simulink model "short_transmission_line_design"  (R2014b)
settings: Solver=ode23tb  StartTime=0.0  StopTime=1  RelTol=1e-3
libraries: powerlib x6, powerlib_meascontrol x6
settings Model: Creator=Amr Saleh  LastModifiedBy=Amr Saleh

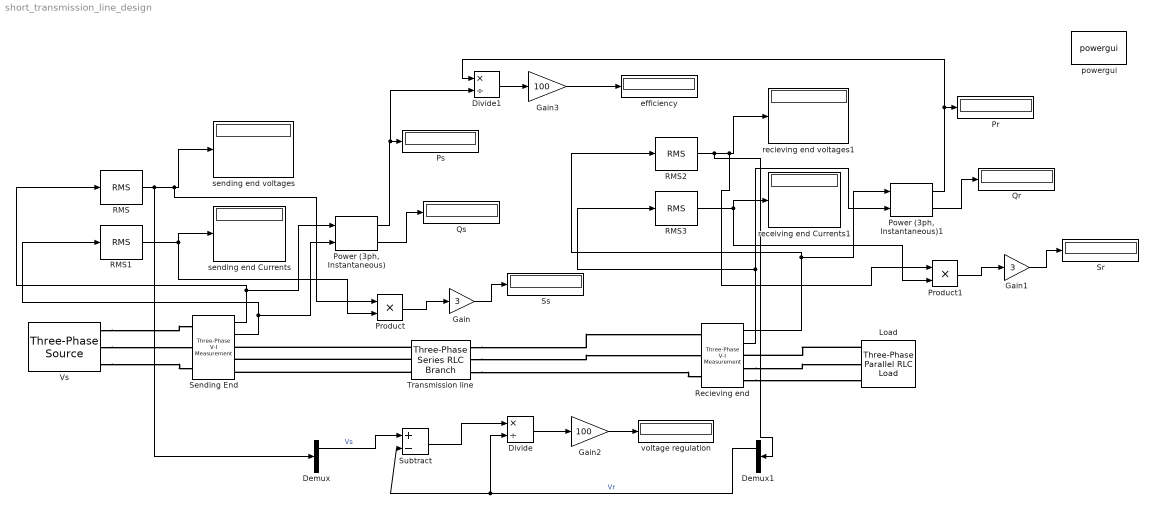
== system short_transmission_line_design ==
  Demux : Demux  Outputs=3
  Demux1 : Demux  Outputs=3
  Divide : Product  Inputs=*/
  Divide1 : Product  Inputs=*/
  Gain : Gain  Gain=3
  Gain1 : Gain  Gain=3
  Gain2 : Gain  Gain=100
  Gain3 : Gain  Gain=100
  Load : powerlib/Elements/Three-Phase Parallel RLC Load  LConnTagsString=A|B|C  Configuration=Y (grounded)  NominalVoltage=220e3  NominalFrequency=60  ActivePower=304.8e6  InductivePower=228.6e6  CapacitivePower=0  Measurements=None  LoadType=constant Z
  "Power (3ph, Instantaneous)" : powerlib_meascontrol/Measurements/Power (3ph, Instantaneous)
  "Power (3ph, Instantaneous)1" : powerlib_meascontrol/Measurements/Power (3ph, Instantaneous)
  Pr : Display
  Product : Product
  Product1 : Product
  Ps : Display
  Qr : Display
  Qs : Display
  RMS{,1..3} (4 alike) : powerlib_meascontrol/Measurements/RMS  TrueRMS=on  Freq=60  RMSInit=0  Ts=0
  Recieving end : powerlib/Measurements/Three-Phase V-I Measurement  VoltageMeasurement=phase-to-ground  SetLabelV=off  LabelV=Vabc  Vpu=off  VpuLL=off  CurrentMeasurement=yes  SetLabelI=off  LabelI=Iabc  Ipu=off  Pbase=100e6  Vbase=500e3  OutputType=Complex  PhasorSimulation=off  PSBequivalent=0
  Sending End : powerlib/Measurements/Three-Phase V-I Measurement  VoltageMeasurement=phase-to-ground  SetLabelV=off  LabelV=Vabc  Vpu=off  VpuLL=off  CurrentMeasurement=yes  SetLabelI=off  LabelI=Iabc  Ipu=off  Pbase=100e6  Vbase=500e3  OutputType=Complex  PhasorSimulation=off  PSBequivalent=0
  Sr : Display
  Ss : Display
  Subtract : Sum  Inputs=+-
  "Transmission line " : powerlib/Elements/Three-Phase Series RLC Branch  LConnTagsString=A|B|C  RConnTagsString=A|B|C  BranchType=RL  Resistance=6  Inductance=0.053052  Capacitance=1e-6  Measurements=None
  Vs : powerlib/Electrical Sources/Three-Phase Source  Voltage=250e3  PhaseAngle=0  Frequency=60  InternalConnection=Yg  SpecifyImpedance=off  Resistance=0  Inductance=0  ShortCircuitLevel=100e6  BaseVoltage=250e3  XRratio=7  BusType=swing  Pref=0  Qref=0  Qmin=-inf  Qmax=inf
  efficiency : Display
  powergui : powerlib/powergui  Priority=1  SimulationMode=Continuous  SolverType=Tustin/Backward Euler (TBE)  SampleTime=50e-6  frequency=60  SPID=off  DisableSnubberDevices=off  DisableRonSwitches=off  DisableVfSwitches=off  SwTol=0  DisplayEquations=off  Interpol=off  methode=off  Ts=100  frequencyindice=60  Pbase=100e6  ErrMax=1e-4  Iterations=50  UnitsV=kV  UnitsW=MW  FunctionMessages=off  echomessages=off  HookPort=off  EnableUseOfTLC=off  x0status=blocks  RestoreLinks=warning  ResistiveCurrentMeasurement=off  Frange=[0:2:500]  Ylog=off  Xlog=on  ShowGrid=off  save=off  variable=ZData  structure=0  ZoomFFT=off  StartTime=0.0  cycles=1  DisplayStyle=1  fundamental=60  FreqAxis=off  MaxFrequency=1000  frequencyindicesteady=1  RmsSteady=1  display=off
  receiving end Currents1 : Display
  recieving end voltages1 : Display
  sending end Currents : Display
  sending end voltages : Display
  voltage regulation : Display
  wires:
  Sending End/1 -> "Power (3ph, Instantaneous)"/1, RMS/1
  RMS/1 -> Demux/1, Product/1, sending end voltages/1
  RMS1/1 -> sending end Currents/1, Product/2
  Sending End/2 -> "Power (3ph, Instantaneous)"/2, RMS1/1
  "Power (3ph, Instantaneous)"/1 -> Divide1/2, Ps/1
  "Power (3ph, Instantaneous)"/2 -> Qs/1
  Product/1 -> Gain/1
  Gain/1 -> Ss/1
  Recieving end/1 -> "Power (3ph, Instantaneous)1"/1, RMS2/1
  RMS2/1 -> Demux1/1, Product1/1, recieving end voltages1/1
  RMS3/1 -> receiving end Currents1/1, Product1/2
  Recieving end/2 -> "Power (3ph, Instantaneous)1"/2, RMS3/1
  "Power (3ph, Instantaneous)1"/1 -> Divide1/1, Pr/1
  "Power (3ph, Instantaneous)1"/2 -> Qr/1
  Product1/1 -> Gain1/1
  Gain1/1 -> Sr/1
  Demux/1 -> Subtract/1  "Vs"
  Demux1/1 -> Divide/2, Subtract/2  "Vr"
  Subtract/1 -> Divide/1
  Divide/1 -> Gain2/1
  Gain2/1 -> voltage regulation/1
  Divide1/1 -> Gain3/1
  Gain3/1 -> efficiency/1
  connections:
  Vs/RConn1 -- Sending End/LConn1
  Vs/RConn2 -- Sending End/LConn2
  Vs/RConn3 -- Sending End/LConn3
  "Transmission line "/LConn1 -- Sending End/RConn1
  "Transmission line "/LConn2 -- Sending End/RConn2
  "Transmission line "/LConn3 -- Sending End/RConn3
  Load/LConn1 -- Recieving end/RConn1
  Recieving end/RConn2 -- Load/LConn2
  Recieving end/RConn3 -- Load/LConn3
  "Transmission line "/RConn1 -- Recieving end/LConn1
  "Transmission line "/RConn2 -- Recieving end/LConn2
  "Transmission line "/RConn3 -- Recieving end/LConn3
